simulink model "bicycle_drift_model_modified"  (R2016a)
settings: Solver=VariableStepAuto  StartTime=0.0  StopTime=15  RelTol=1e-3
values from neighbouring files (symbols this model uses):
  a = 0.1329    [dynamics.m]    (also in setup.m; tire_test.m = 0.11372)
  b = 0.1221    [dynamics.m]    (also in setup.m; tire_test.m = 0.14328)
  C_alpha = 120000    [dynamics.m]    (also in setup.m = 1200; tire_test.m = 197)
  initial_states = [0 0 0.1]    [setup.m]
  Iz = 0.020899525    [dynamics.m]    (also in setup.m; tire_test.m = 0.025)
  L = 0.255    [dynamics.m]    (also in setup.m; tire_test.m = 0.257; veh_object2.m = obj_length)
  m = 2.622    [dynamics.m]    (also in setup.m; tire_test.m = 2.35)
  mu = 0.37    [dynamics.m]    (also in setup.m; tire_test.m = 1.31)
undefined symbols (not defined in the file): animation_update_interval, datetime, enable_CG_trace, enable_rearAxle_trace, plotAxisLimitMode, plotAxisLimits, save_anim_frames, vehicle_length, vehicle_width
settings Model: Creator=Cyrus  LastModifiedBy=Cyrus

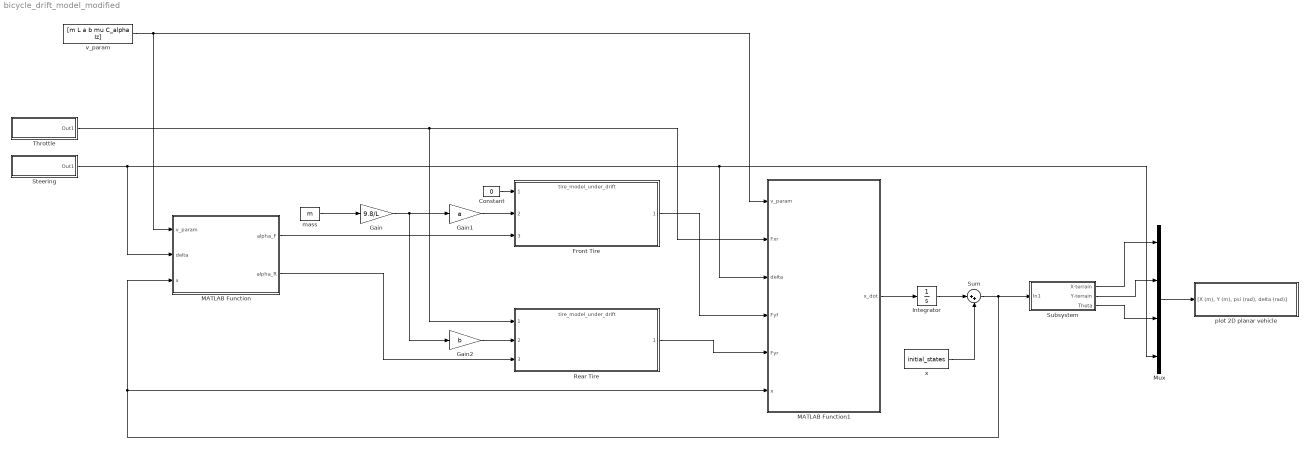
== system bicycle_drift_model_modified ==
  Constant : Constant  Value=0
  Front Tire : ModelReference  ModelNameDialog=tire_model_under_drift.slx  SimulationMode=Normal  ModelReferenceVersion=1.22
  Gain : Gain  Gain=9.8/L
  Gain1 : Gain  Gain=a
  Gain2 : Gain  Gain=b
  Integrator : Integrator
  MATLAB Function : MATLAB Function  TreatAsAtomicUnit=on
  MATLAB Function1 : MATLAB Function  TreatAsAtomicUnit=on
  Mux : Mux
  Rear Tire : ModelReference  ModelNameDialog=tire_model_under_drift.slx  SimulationMode=Normal  ModelReferenceVersion=1.22
  Steering : Subsystem
  Subsystem : Subsystem
  Sum : Sum  Inputs=|++
  Throttle : Subsystem
  mass : Constant  Value=m
  plot 2D planar vehicle : Subsystem  mask(6DoF Animation){axisMode=plotAxisLimitMode, ax=plotAxisLimits, Ts=animation_update_interval, enable_CG_trace=enable_CG_trace, enable_rearAxle_trace=enable_rearAxle_trace, save_anim_frames=save_anim_frames, anim_frame_name_str=char(datetime('now','Format','yyyy-MM-dd_HH_mm_ss')), L=vehicle_length, W=vehicle_width}
      mask prompts: axisMode "Axis Mode (0->auto, 1->fixed, BOTH use Axes Limits below)"; ax "Axes limits [xmin xmax ymin ymax] (m):"; Ts "Time interval between updates (s):"; enable_CG_trace "Enable vehicle CG trace? (0/1)"; enable_rearAxle_trace "Enable rear axle trace? (0/1)"; save_anim_frames "Save animaton frames? (0/1)"; anim_frame_name_str "Animation sequence name (if save frames==1)"; L "Vehicle length (m)"; W "Vehicle width (m)"
      mask help:
      | Create a 2D animated view of a steering vehicle model with tires.
      |
      | Marc Compere
      | CompereM@saic.com
      | created : 22 August 2002
      | modified: 28 Dec 2015
      mask init:
      | Config.axisMode=axisMode;
      | Config.ax=ax;
      | Config.Ts=Ts;
      | Config.enable_CG_trace=enable_CG_trace;
      | Config.enable_rearAxle_trace=enable_rearAxle_trace;
      | Config.save_anim_frames=save_anim_frames;
      | Config.anim_frame_name_str=anim_frame_name_str;
      | Config.L=L;
      | Config.W=W;
      mask Help:
      | <p>This block generates a 3 dimensional display of a simulation trajectory, with the craft orientation displayed during flight</p>
      | 
      | <p>There are two inputs to this block, Position and Euler.  These inputs contain more than one signal as described below.</p>
      | 
      | <p><H4>Block Vector Input - Position</H4>
      | <ul>
      | <li>X Position</li>
      | <li>Y Position</li>
      | <li>Z Position</li>
      | </ul>
      | </p>
      | 
      | <p><H4>Block Vector Input - Euler</H4>
      |     <ul>
      |     <li>Roll Attitude</li>
      |     <li>Pitch Attitude</li>
      |     <li>Yaw Attitude</li>
      |    </ul>
      |    </p>
  v_param : Constant  Value=[m L a b mu C_alpha Iz]
  x : Constant  Value=initial_states
  wires:
  mass/1 -> Gain/1
  Gain1/1 -> Front Tire/2
  Gain2/1 -> Rear Tire/2
  MATLAB Function/1(alpha_F) -> Front Tire/3
  MATLAB Function/2(alpha_R) -> Rear Tire/3
  Gain/1 -> Gain2/1, Gain1/1
  Sum/1 -> MATLAB Function/3(x), MATLAB Function1/6(x), Subsystem/1(In1)
  MATLAB Function1/1(x_dot) -> Integrator/1
  Front Tire/1 -> MATLAB Function1/4(Fyf)
  Rear Tire/1 -> MATLAB Function1/5(Fyr)
  Constant/1 -> Front Tire/1
  Integrator/1 -> Sum/1
  x/1 -> Sum/2
  Steering/1(Out1) -> Mux/4, MATLAB Function1/3(delta), MATLAB Function/2(delta)
  Subsystem/1(X-terrain) -> Mux/1
  Subsystem/2(Y-terrain) -> Mux/2
  Subsystem/3("Theta ") -> Mux/3
  Mux/1 -> plot 2D planar vehicle/1("[X (m), Y (m), psi (rad), delta (rad)]")
  v_param/1 -> MATLAB Function1/1(v_param), MATLAB Function/1(v_param)
  Throttle/1(Out1) -> Rear Tire/1, MATLAB Function1/2(Fxr)

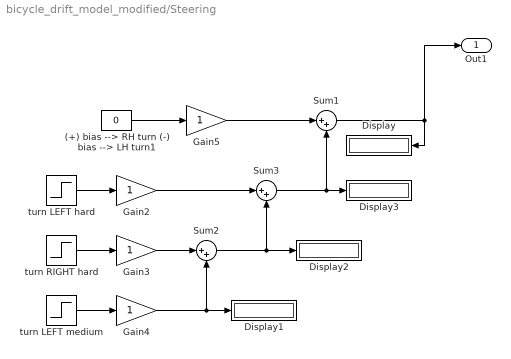
== system bicycle_drift_model_modified/Steering ==
  (+) bias --> RH turn (-) bias --> LH turn1 : Constant  Value=0
  Display{,1..3} (4 alike) : Display
  Gain{2..5} (4 alike) : Gain
  Sum1 : Sum  Inputs=|++
  Sum2 : Sum  Inputs=|++
  Sum3 : Sum  Inputs=|++
  turn LEFT hard : Step  Time=0.5  After=-0.5  SampleTime=0
  turn LEFT medium : Step  Time=11  After=-0.5  SampleTime=0
  turn RIGHT hard : Step  Time=6  After=+1  SampleTime=0
  Out1 : Outport
  wires:
  Sum1/1 -> Out1/1, Display/1
  (+) bias --> RH turn (-) bias --> LH turn1/1 -> Gain5/1
  turn RIGHT hard/1 -> Gain3/1
  turn LEFT medium/1 -> Gain4/1
  turn LEFT hard/1 -> Gain2/1
  Sum2/1 -> Display2/1, Sum3/2
  Sum3/1 -> Display3/1, Sum1/2
  Gain2/1 -> Sum3/1
  Gain3/1 -> Sum2/1
  Gain4/1 -> Display1/1, Sum2/2
  Gain5/1 -> Sum1/1

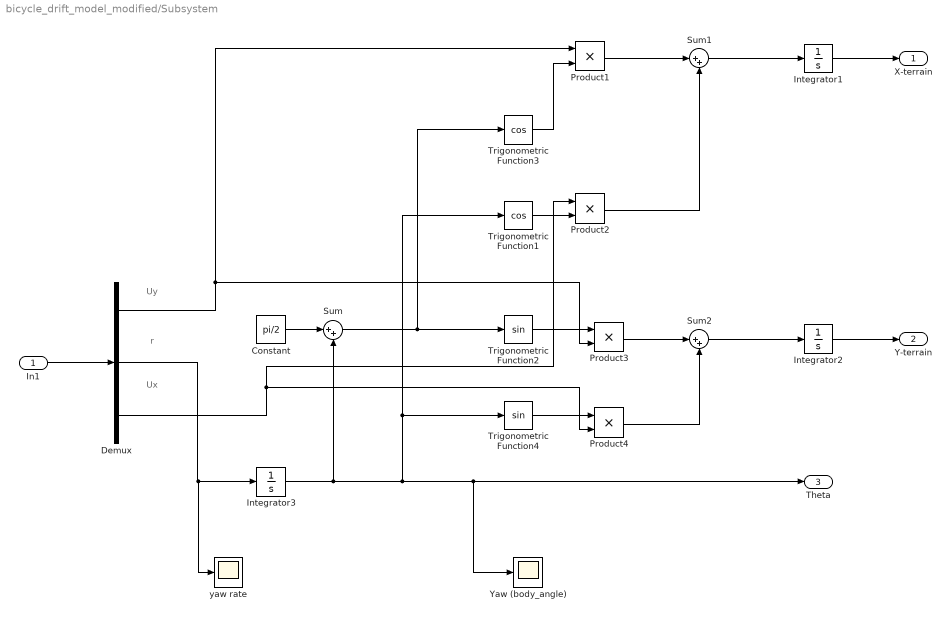
== system bicycle_drift_model_modified/Subsystem ==
  note: r
  note: Ux
  note: Uy
  In1 : Inport
  Constant : Constant  Value=pi/2
  Demux : Demux  Outputs=3
  Integrator1 : Integrator
  Integrator2 : Integrator
  Integrator3 : Integrator
  Product{1..4} (4 alike) : Product
  Sum : Sum  Inputs=|++
  Sum1 : Sum  Inputs=|++
  Sum2 : Sum  Inputs=|++
  Trigonometric Function1 : Trigonometry  Operator=cos
  Trigonometric Function2 : Trigonometry
  Trigonometric Function3 : Trigonometry  Operator=cos
  Trigonometric Function4 : Trigonometry
  Yaw (body_angle) : Scope
  yaw rate : Scope
  X-terrain : Outport
  Y-terrain : Outport  Port=2
  "Theta " : Outport  Port=3
  wires:
  In1/1 -> Demux/1
  Demux/2 -> yaw rate/1, Integrator3/1
  Integrator3/1 -> Sum/2, Trigonometric Function4/1, Trigonometric Function1/1, "Theta "/1, Yaw (body_angle)/1
  Sum/1 -> Trigonometric Function2/1, Trigonometric Function3/1
  Constant/1 -> Sum/1
  Trigonometric Function3/1 -> Product1/2
  Demux/1 -> Product1/1, Product3/2
  Trigonometric Function1/1 -> Product2/2
  Demux/3 -> Product4/2, Product2/1
  Trigonometric Function4/1 -> Product4/1
  Trigonometric Function2/1 -> Product3/1
  Product1/1 -> Sum1/1
  Product2/1 -> Sum1/2
  Sum1/1 -> Integrator1/1
  Integrator1/1 -> X-terrain/1
  Product3/1 -> Sum2/1
  Product4/1 -> Sum2/2
  Sum2/1 -> Integrator2/1
  Integrator2/1 -> Y-terrain/1

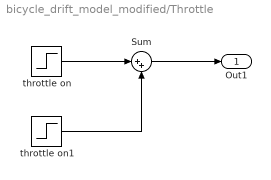
== system bicycle_drift_model_modified/Throttle ==
  Sum : Sum  Inputs=|++
  throttle on : Step  Time=0  SampleTime=0
  throttle on1 : Step  Time=6  After=0  SampleTime=0
  Out1 : Outport
  wires:
  throttle on1/1 -> Sum/2
  throttle on/1 -> Sum/1
  Sum/1 -> Out1/1

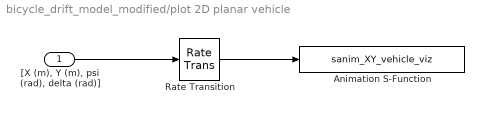
== system bicycle_drift_model_modified/plot 2D planar vehicle ==
  "[X (m), Y (m), psi (rad), delta (rad)]" : Inport
  Animation S-Function : S-Function  FunctionName=sanim_XY_vehicle_viz  Parameters=Config  SFunctionDeploymentMode=off  EnableBusSupport=off
  Rate Transition : RateTransition  Integrity=off
  wires:
  "[X (m), Y (m), psi (rad), delta (rad)]"/1 -> Rate Transition/1
  Rate Transition/1 -> Animation S-Function/1

== matlab function bicycle_drift_model_modified/MATLAB Function1 ==
  data: v_param input; Fxr input; delta input; Fyf input; Fyr input; x_dot output; x input
function x_dot = fcn(v_param,Fxr,delta,Fyf,Fyr,x)
%#codegen
m = v_param(1);
a = v_param(3);
b = v_param(4);
Iz = v_param(7);

Uy = x(1);
r = x(2);
Ux = x(3);

Uy_dot = (Fyf*cos(delta)+Fyr)/m-r*Ux;
r_dot = (a*Fyf*cos(delta)-b*Fyr)/Iz;
Ux_dot = (Fxr-Fyf*sin(delta))/m+r*Uy;

x_dot = [Uy_dot r_dot Ux_dot];

== matlab function bicycle_drift_model_modified/MATLAB Function ==
  data: v_param input; delta input; x input; alpha_F output; alpha_R output
function [alpha_F, alpha_R] = fcn(v_param,delta,x)
%#codegen
a = v_param(3);
b = v_param(4);

Uy = x(1);
r = x(2);
Ux = x(3);

alpha_F = atan((Uy+a*r)/Ux)-delta;
alpha_R = atan((Uy-b*r)/Ux);
